simulink model "Practica32022A"  (R2022a)
settings: Solver=FixedStepDiscrete  StartTime=0.0  StopTime=10  FixedStep=0.001  RelTol=1e-3
settings Model: Creator=edgar  LastModifiedBy=edgar
settings ModelReferenceCC: EnableRefExpFcnMdlSchedulingChecks=off
settings RTWCC: Description=Generic Real-Time Target

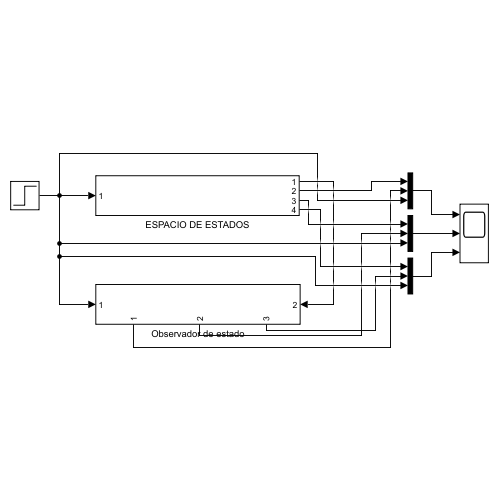
[thumbnail: Simulink's stored preview of the top-level diagram]
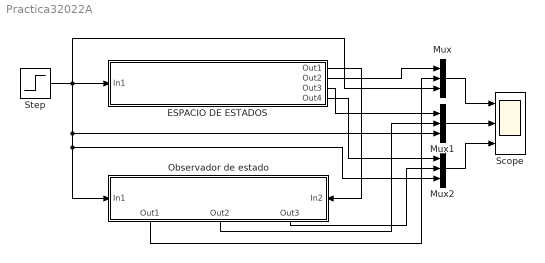
== system Practica32022A ==
  ESPACIO DE ESTADOS : Subsystem
  Mux : Mux  Inputs=3
  Mux1 : Mux  Inputs=3
  Mux2 : Mux  Inputs=3
  Observador de estado : Subsystem
      settings: PortSchema="{\"entries\":[{\"content\":{\"sides\":[{\"content\":{\"connectorIds\":[\"In1\"]},\"type\":\"ConnectorPlacement.EquallySpacedRectSide\",\"uuid\":\"9933af09-e30a-4a3c-a0e3-dffec2223d50\"},{\"content\":{\"connectorIds\":[\"In2\"],\"side\":\"RIGHT\"},\"type\":\"ConnectorPlacement.EquallySpacedRectSide\",\"uuid\":\"a5fb4d5c-b0b2-4fa6-9ed9-ad5917edf078\"},{\"content\":{\"side\":\"TOP\"},\"type\":\"ConnectorPlacement.EquallySpacedRectSide\",\"uuid\":\"6702ee26-218a-4e5a-8b7f-2d20323f3f9e\"},{\"content\":{\"connectorIds\":[\"Out1\",\"Out2\",\"Out3\"],\"side\":\"BOTTOM\"},\"type\":\"ConnectorPlacement.EquallySpacedRectSide\",\"uuid\":\"bb15bb68-788c-4e99-a02f-77e7536579be\"}]},\"type\":\"ConnectorPlacement.EquallySpacedConnector\",\"uuid\":\"78becabe-a2b6-43cf-81c2-35f37bc38762\"}],\"packageUris\":[\"http://schema.mathworks.com/mf0/Connector/R2020b\"],\"version\":\"1.0\"}"
  Scope : Scope  NumInputPorts=3
  Step : Step  Time=0  SampleTime=0
  wires:
  Step/1 -> Mux2/3, Observador de estado/1(In1), Mux1/3, Mux/3, ESPACIO DE ESTADOS/1(In1)
  ESPACIO DE ESTADOS/1(Out1) -> Observador de estado/2(In2)
  Mux/1 -> Scope/1
  Mux1/1 -> Scope/2
  Mux2/1 -> Scope/3
  ESPACIO DE ESTADOS/2(Out2) -> Mux/1
  Observador de estado/1(Out1) -> Mux/2
  Observador de estado/2(Out2) -> Mux1/2
  Observador de estado/3(Out3) -> Mux2/2
  ESPACIO DE ESTADOS/3(Out3) -> Mux1/1
  ESPACIO DE ESTADOS/4(Out4) -> Mux2/1

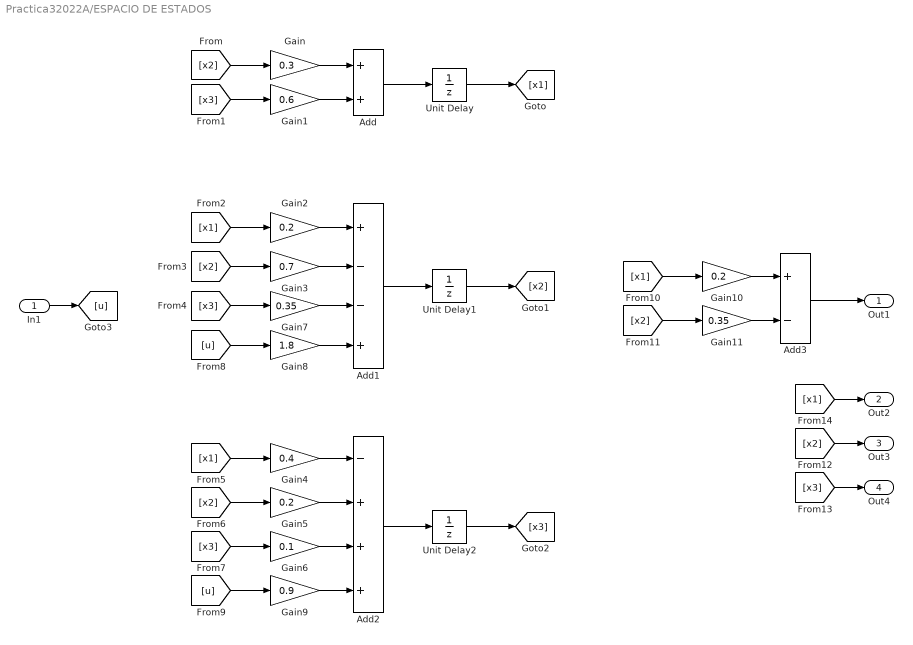
== system Practica32022A/ESPACIO DE ESTADOS ==
  In1 : Inport
  Add : Sum
  Add1 : Sum  Inputs=+--+
  Add2 : Sum  Inputs=-+++
  Add3 : Sum  Inputs=+-
  Gain : Gain  Gain=0.3
  Gain1 : Gain  Gain=0.6
  Gain10 : Gain  Gain=0.2
  Gain11 : Gain  Gain=0.35
  Gain2 : Gain  Gain=0.2
  Gain3 : Gain  Gain=0.7
  Gain4 : Gain  Gain=0.4
  Gain5 : Gain  Gain=0.2
  Gain6 : Gain  Gain=0.1
  Gain7 : Gain  Gain=0.35
  Gain8 : Gain  Gain=1.8
  Gain9 : Gain  Gain=0.9
  Unit Delay : UnitDelay  InitialCondition=1  SampleTime=-1  HasFrameUpgradeWarning=on
  Unit Delay1 : UnitDelay  InitialCondition=2  SampleTime=-1  HasFrameUpgradeWarning=on
  Unit Delay2 : UnitDelay  InitialCondition=3  SampleTime=-1  HasFrameUpgradeWarning=on
  Out1 : Outport
  Out2 : Outport  Port=2
  Out3 : Outport  Port=3
  Out4 : Outport  Port=4
  wires:
  Unit Delay/1 -> [x1]
  Unit Delay1/1 -> [x2]
  Unit Delay2/1 -> [x3]
  Add2/1 -> Unit Delay2/1
  Add1/1 -> Unit Delay1/1
  Add/1 -> Unit Delay/1
  Gain/1 -> Add/1
  Gain1/1 -> Add/2
  Gain7/1 -> Add1/3
  Gain3/1 -> Add1/2
  Gain2/1 -> Add1/1
  Gain5/1 -> Add2/2
  Gain4/1 -> Add2/1
  Gain6/1 -> Add2/3
  [x2] -> Gain/1
  [x3] -> Gain1/1
  [x1] -> Gain2/1
  [x2] -> Gain3/1
  [x3] -> Gain7/1
  [x1] -> Gain4/1
  [x2] -> Gain5/1
  [x3] -> Gain6/1
  In1/1 -> [u]
  Gain9/1 -> Add2/4
  [u] -> Gain9/1
  [u] -> Gain8/1
  Gain8/1 -> Add1/4
  Add3/1 -> Out1/1
  [x2] -> Gain11/1
  [x1] -> Gain10/1
  Gain11/1 -> Add3/2
  Gain10/1 -> Add3/1
  [x2] -> Out3/1
  [x3] -> Out4/1
  [x1] -> Out2/1

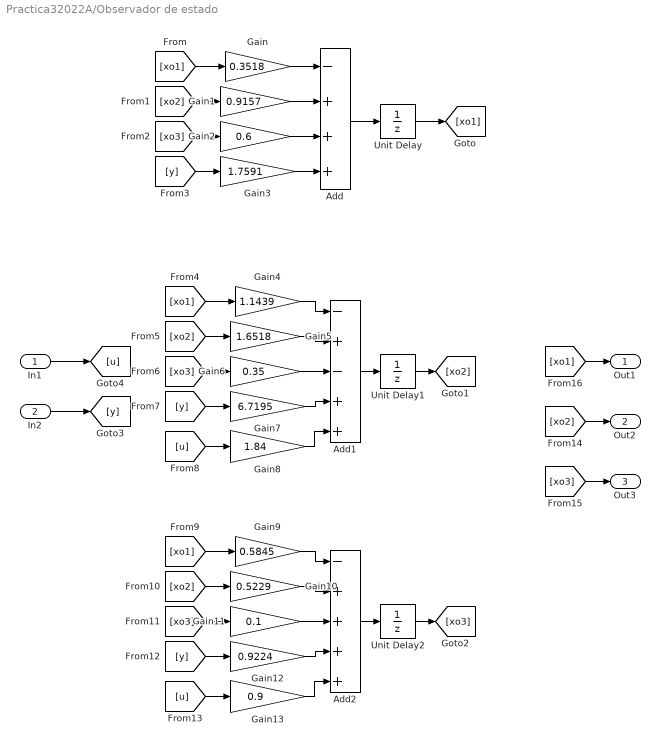
== system Practica32022A/Observador de estado ==
  In1 : Inport
  In2 : Inport  Port=2
  Add : Sum  Inputs=-+++
  Add1 : Sum  Inputs=-+-++
  Add2 : Sum  Inputs=-++++
  Gain : Gain  Gain=0.3518
  Gain1 : Gain  Gain=0.9157
  Gain10 : Gain  Gain=0.5229
  Gain11 : Gain  Gain=0.1
  Gain12 : Gain  Gain=0.9224
  Gain13 : Gain  Gain=0.9
  Gain2 : Gain  Gain=0.6
  Gain3 : Gain  Gain=1.7591
  Gain4 : Gain  Gain=1.1439
  Gain5 : Gain  Gain=1.6518
  Gain6 : Gain  Gain=0.35
  Gain7 : Gain  Gain=6.7195
  Gain8 : Gain  Gain=1.84
  Gain9 : Gain  Gain=0.5845
  Unit Delay : UnitDelay  InitialCondition=5  SampleTime=-1  HasFrameUpgradeWarning=on
  Unit Delay1 : UnitDelay  InitialCondition=-2  SampleTime=-1  HasFrameUpgradeWarning=on
  Unit Delay2 : UnitDelay  InitialCondition=-4  SampleTime=-1  HasFrameUpgradeWarning=on
  Out1 : Outport
  Out2 : Outport  Port=2
  Out3 : Outport  Port=3
  wires:
  Unit Delay/1 -> [xo1]
  Unit Delay1/1 -> [xo2]
  Unit Delay2/1 -> [xo3]
  In2/1 -> [y]
  In1/1 -> [u]
  Add/1 -> Unit Delay/1
  Gain/1 -> Add/1
  Gain3/1 -> Add/4
  Gain2/1 -> Add/3
  Gain1/1 -> Add/2
  [xo1] -> Gain/1
  [xo2] -> Gain1/1
  [xo3] -> Gain2/1
  [y] -> Gain3/1
  [xo2] -> Gain5/1
  Gain5/1 -> Add1/2
  Gain6/1 -> Add1/3
  Gain7/1 -> Add1/4
  [xo1] -> Gain4/1
  Gain4/1 -> Add1/1
  [y] -> Gain7/1
  [xo3] -> Gain6/1
  Add1/1 -> Unit Delay1/1
  Gain8/1 -> Add1/5
  [u] -> Gain8/1
  [u] -> Gain13/1
  Gain13/1 -> Add2/5
  [xo3] -> Gain11/1
  [y] -> Gain12/1
  Gain9/1 -> Add2/1
  [xo1] -> Gain9/1
  Gain12/1 -> Add2/4
  Gain11/1 -> Add2/3
  Gain10/1 -> Add2/2
  [xo2] -> Gain10/1
  Add2/1 -> Unit Delay2/1
  [xo2] -> Out2/1
  [xo3] -> Out3/1
  [xo1] -> Out1/1
